simulink model "sim_pos_dist_obs_tcyb"  (R2020a)
settings: Solver=ode4  StartTime=0.0  StopTime=30.0  FixedStep=0.01  RelTol=1e-3
values from neighbouring files (symbols this model uses):
  alfa_theta = 20    [draw_compare_dist_pos_obs.m]
  alfa_theta_obs = 100    [draw_compare_dist_pos_obs.m]
  beta1 = 1.2    [draw_compare_dist_pos_obs.m]
  beta2 = 0.8    [draw_compare_dist_pos_obs.m]
  delta_p_i_0 = zeros(3, NF)    [draw_compare_dist_pos_obs.m]
  delta_v_i_0 = zeros(3, NF)    [draw_compare_dist_pos_obs.m]
  dp_aa_t = 0.2 * ones(3, 5) + ( 1.0 - 0.2 ) * rand(3, 5)    [draw_compare_dist_pos_obs.m]
  dp_ff_t = [ 0.4 * ones(1, 5) + ( 1.0 - 0.4 ) * rand(1, 5);                      0.4 * ones(1, 5) + ( 1.0 - 0.4 ) * rand(1, 5);                      0.2 * ones(1, 5) + ( 0.6 - 0.2 ) * rand(1, 5) ]    [draw_compare_dist_pos_obs.m]
  dp_phi_t = ( - pi / 2 ) * ones(3, 5) + ( pi / 2 - ( - pi / 2 ) ) * rand(3, 5)    [draw_compare_dist_pos_obs.m]
  eps_zeta = 0.2    [draw_compare_dist_pos_obs.m]
  etai_0 = zeros(3,5)    [draw_compare_dist_pos_obs.m]
  gamma_obs_1 = 4    [draw_compare_dist_pos_obs.m]
  gamma_obs_2 = 4    [draw_compare_dist_pos_obs.m]
  kai_1_t = 0.02    [draw_compare_dist_pos_obs.m]
  kai_3_t = 0.1    [draw_compare_dist_pos_obs.m]
  kai_chi_1 = diag([6; 6; 6])    [draw_compare_dist_pos_obs.m]
  kai_chi_2 = diag([6; 6; 6])    [draw_compare_dist_pos_obs.m]
  kai_u_1 = diag([8; 8; 8])    [draw_compare_dist_pos_obs.m]
  kai_u_2 = diag([8; 8; 8])    [draw_compare_dist_pos_obs.m]
  ksii_0 = zeros(3,5)    [draw_compare_dist_pos_obs.m]
  l1v = diag([20; 20; 20])    [draw_compare_dist_pos_obs.m]
  l2v = diag([30; 30; 30])    [draw_compare_dist_pos_obs.m]
  mass_i = zeros(1,NF)    [draw_compare_dist_pos_obs.m]
  Mii = diag([1;0;0;0;1])    [draw_compare_dist_pos_obs.m]
  pos0 = zeros(3, 1)    [draw_compare_dist_pos_obs.m]
  PZ0 = P0(3)    [draw_compare_dist_pos_obs.m]
  PZ1 = 10    [draw_compare_dist_pos_obs.m]
  Qci_init = repmat([1;0;0;0],1,NF)    [draw_compare_dist_pos_obs.m]
  R0 = 4    [draw_compare_dist_pos_obs.m]
  R1 = 8    [draw_compare_dist_pos_obs.m]
  Rx2 = 10    [draw_compare_dist_pos_obs.m]
  Ry2 = 6    [draw_compare_dist_pos_obs.m]
  Rz2 = 4    [draw_compare_dist_pos_obs.m]
  T0 = 0    [draw_compare_dist_pos_obs.m]
  T1 = tseq1    (= 10)    [draw_compare_dist_pos_obs.m]
  T12 = tseq1 + tseq12    (= 20)    [draw_compare_dist_pos_obs.m]
  T2 = tseq1 + tseq12 + tseq2    (= 30)    [draw_compare_dist_pos_obs.m]
  tf2_zeta = 2    [draw_compare_dist_pos_obs.m]
  theta0 = ( 2 / 5 ) * pi    (= 1.25663706144)    [draw_compare_dist_pos_obs.m]
  vel0 = zeros(3, 1)    [draw_compare_dist_pos_obs.m]
  Wij = [0,0,1,0,0;              0,0,1,1,0;              1,0,0,0,1;              0,1,1,0,0;              0,0,1,0,0]    [draw_compare_dist_pos_obs.m]
  X1 = 8    [draw_compare_dist_pos_obs.m]
  X2 = 2    [draw_compare_dist_pos_obs.m]
  X3 = 3    [draw_compare_dist_pos_obs.m]
  Y1 = 10    [draw_compare_dist_pos_obs.m]
  Y2 = 2    [draw_compare_dist_pos_obs.m]
  Y3 = 4    [draw_compare_dist_pos_obs.m]
  Z1 = 4    [draw_compare_dist_pos_obs.m]
  Z2 = -6    [draw_compare_dist_pos_obs.m]
  Z3 = 2    [draw_compare_dist_pos_obs.m]
undefined symbols (not defined in the file or in its folder): cal_frac_squ, p_beta1, p_beta2, p_dbeta1, p_dbeta2, p_gamma1_pos, p_gamma1_vel, p_gamma2_pos, p_gamma2_vel, q_beta1, q_beta2, q_dbeta1, q_dbeta2, q_gamma1_pos, q_gamma1_vel, q_gamma2_pos, q_gamma2_vel
(part 2 of 4)

== matlab function sim_pos_dist_obs_tcyb/choose ksi_est_err 19 ==
  data: x input; y output
function y = fcn(x)
iiuav = 5;
y = x(:,iiuav);

== matlab function sim_pos_dist_obs_tcyb/leader control input ==
  data: t input; u0 output; T1 input; T2 input; R0 input; R1 input; Rx2 input; Ry2 input; Rz2 input
function u0  = fcn(t, T1, T2, R0, R1, Rx2, Ry2, Rz2)
%%%% 给出领导者参考加速度控制输入
u0 = zeros(3, 1);

if t <= ( T1 + 1e-05 )
    u0(1, 1) = - ( 4 * pi * sin( ( 2 * pi * ( t - 0 ) ) / ( 0 - T1 ) ) * ( R0 - R1 ) ) / ( ( 0 - T1 ) ^ 2 ) ...
                        - ( 4 * ( pi ^ 2 ) * cos( ( 2 * pi * ( t - 0 ) ) / ( 0 - T1 ) ) ...
                        * ( R0 + ( ( R0 - R1 ) * ( t - 0 ) ) / ( 0 - T1 ) ) ) / ( ( 0 - T1 ) ^ 2 );
    u0(2, 1) = ( 4 * pi * cos( ( 2 * pi * ( t - 0 ) ) / ( 0 - T1 ) ) * ( R0 - R1 ) ) / ( ( 0 - T1 ) ^ 2 ) ...
                        - ( 4 * ( pi ^ 2 ) * sin( ( 2 * pi * ( t - 0 ) ) / ( 0 - T1 ) ) ...
                        * ( R0 + ( ( R0 - R1 ) * ( t - 0 ) ) / ( 0 - T1 ) ) ) / ( ( 0 - T1 ) ^ 2 );
    u0(3, 1) = 0;
else
    u0(1, 1) = ( 4 * Rx2 * ( pi ^ 2 ) * cos( ( 2 * pi * ( t - T1 ) ) / ( T1 - T2 ) ) ) / ( ( T1 - T2 ) ^ 2 );
    u0(2, 1) = - ( 16 * Ry2 * ( pi ^ 2 ) * sin( ( 4 * pi * ( t - T1 ) ) / ( T1 - T2 ) ) ) / ( ( T1 - T2 ) ^ 2 );
    u0(3, 1) = ( 16 * Rz2 * ( pi ^ 2 ) * sin( ( 4 * pi * ( t - T1 ) ) / ( T1 - T2 ) ) ) / ( ( T1 - T2 ) ^ 2 );
end

== matlab function sim_pos_dist_obs_tcyb/choose ksi_est_err 20 ==
  data: x input; y output
function y = fcn(x)
iiuav = 5;
y = x(:,iiuav);

== matlab function sim_pos_dist_obs_tcyb/trans to column18 ==
  data: x input; y output
function y = fcn(x)
y = x(:);

== matlab function sim_pos_dist_obs_tcyb/trans to column19 ==
  data: x input; y output
function y = fcn(x)
y = x(:);

== matlab function sim_pos_dist_obs_tcyb/cal dchi agent 1 ==
  data: kai_chi_1 input; d_chi_1 output; kai_chi_2 input; d_theta_err_ksi_1_vec input; d_theta_err_ksi_2_vec input
function d_chi_1 = fcn(kai_chi_1, kai_chi_2, d_theta_err_ksi_1_vec, d_theta_err_ksi_2_vec)
%%%% 固定时间虚拟速度控制量导数d_chi
iiuav = 1;
d_chi_1 = -kai_chi_1 * d_theta_err_ksi_1_vec(:,iiuav) - kai_chi_2 * d_theta_err_ksi_2_vec(:,iiuav);

== matlab function sim_pos_dist_obs_tcyb/combine dtheta_err_ksi ==
  data: d_theta_err_ksi_1_1 input; d_theta_err_ksi_1_2 input; d_theta_err_ksi_1_3 input; d_theta_err_ksi_1_4 input; d_theta_err_ksi_1_5 input; d_theta_err_ksi_1_vec output; d_theta_err_ksi_2_1 input; d_theta_err_ksi_2_vec output; d_theta_err_ksi_2_2 input; d_theta_err_ksi_2_3 input; d_theta_err_ksi_2_4 input; d_theta_err_ksi_2_5 input
function [d_theta_err_ksi_1_vec, d_theta_err_ksi_2_vec]  = fcn(d_theta_err_ksi_1_1, d_theta_err_ksi_1_2, d_theta_err_ksi_1_3, d_theta_err_ksi_1_4, d_theta_err_ksi_1_5, ...
                                                                                                                d_theta_err_ksi_2_1, d_theta_err_ksi_2_2, d_theta_err_ksi_2_3, d_theta_err_ksi_2_4, d_theta_err_ksi_2_5)
%%%% 合并平滑函数的导数
d_theta_err_ksi_1_vec = [d_theta_err_ksi_1_1(:), d_theta_err_ksi_1_2(:), d_theta_err_ksi_1_3(:), d_theta_err_ksi_1_4(:), d_theta_err_ksi_1_5(:)];
d_theta_err_ksi_2_vec = [d_theta_err_ksi_2_1(:), d_theta_err_ksi_2_2(:), d_theta_err_ksi_2_3(:), d_theta_err_ksi_2_4(:), d_theta_err_ksi_2_5(:)];

== matlab function sim_pos_dist_obs_tcyb/cal dchi agent 2 ==
  data: kai_chi_1 input; d_chi_2 output; kai_chi_2 input; d_theta_err_ksi_1_vec input; d_theta_err_ksi_2_vec input
function d_chi_2 = fcn(kai_chi_1, kai_chi_2, d_theta_err_ksi_1_vec, d_theta_err_ksi_2_vec)
%%%% 固定时间虚拟速度控制量导数d_chi
iiuav = 2;
d_chi_2 = -kai_chi_1 * d_theta_err_ksi_1_vec(:,iiuav) - kai_chi_2 * d_theta_err_ksi_2_vec(:,iiuav);

== matlab function sim_pos_dist_obs_tcyb/cal dchi agent 3 ==
  data: kai_chi_1 input; d_chi_3 output; kai_chi_2 input; d_theta_err_ksi_1_vec input; d_theta_err_ksi_2_vec input
function d_chi_3 = fcn(kai_chi_1, kai_chi_2, d_theta_err_ksi_1_vec, d_theta_err_ksi_2_vec)
%%%% 固定时间虚拟速度控制量导数d_chi
iiuav = 3;
d_chi_3 = -kai_chi_1 * d_theta_err_ksi_1_vec(:,iiuav) - kai_chi_2 * d_theta_err_ksi_2_vec(:,iiuav);

== matlab function sim_pos_dist_obs_tcyb/cal dchi agent 4 ==
  data: kai_chi_1 input; d_chi_4 output; kai_chi_2 input; d_theta_err_ksi_1_vec input; d_theta_err_ksi_2_vec input
function d_chi_4 = fcn(kai_chi_1, kai_chi_2, d_theta_err_ksi_1_vec, d_theta_err_ksi_2_vec)
%%%% 固定时间虚拟速度控制量导数d_chi
iiuav = 4;
d_chi_4 = -kai_chi_1 * d_theta_err_ksi_1_vec(:,iiuav) - kai_chi_2 * d_theta_err_ksi_2_vec(:,iiuav);

== matlab function sim_pos_dist_obs_tcyb/cal dchi agent 5 ==
  data: kai_chi_1 input; d_chi_5 output; kai_chi_2 input; d_theta_err_ksi_1_vec input; d_theta_err_ksi_2_vec input
function d_chi_5 = fcn(kai_chi_1, kai_chi_2, d_theta_err_ksi_1_vec, d_theta_err_ksi_2_vec)
%%%% 固定时间虚拟速度控制量导数d_chi
iiuav = 5;
d_chi_5 = -kai_chi_1 * d_theta_err_ksi_1_vec(:,iiuav) - kai_chi_2 * d_theta_err_ksi_2_vec(:,iiuav);

== matlab function sim_pos_dist_obs_tcyb/combine dchi ==
  data: d_chi_1 input; d_chi_2 input; d_chi_3 input; d_chi_4 input; d_chi_5 input; d_chi_vec output
function d_chi_vec  = fcn(d_chi_1, d_chi_2, d_chi_3, d_chi_4, d_chi_5)
%%%% 合并领导者位置观测器输出结果
d_chi_vec = [d_chi_1(:), d_chi_2(:), d_chi_3(:), d_chi_4(:), d_chi_5(:)];

== matlab function sim_pos_dist_obs_tcyb/cal x1_hat agent 4 ==
  data: gamma_obs_1 input; zeta2 input; d_x1_hat_4 output; dzeta2 input; x2_hat_vec input; x1_tilt_vec input
function d_x1_hat_4 = fcn(gamma_obs_1, zeta2, dzeta2, x2_hat_vec, x1_tilt_vec)
%%%% 计算状态观测误差
iiuav = 4;
d_x1_hat_4 = x2_hat_vec(:,iiuav) + gamma_obs_1 * zeta2 * x1_tilt_vec(:,iiuav) + ( 2 * dzeta2 / zeta2 ) * x1_tilt_vec(:,iiuav);

== matlab function sim_pos_dist_obs_tcyb/cal x1_hat agent 5 ==
  data: gamma_obs_1 input; zeta2 input; d_x1_hat_5 output; dzeta2 input; x2_hat_vec input; x1_tilt_vec input
function d_x1_hat_5 = fcn(gamma_obs_1, zeta2, dzeta2, x2_hat_vec, x1_tilt_vec)
%%%% 计算状态观测误差
iiuav = 5;
d_x1_hat_5 = x2_hat_vec(:,iiuav) + gamma_obs_1 * zeta2 * x1_tilt_vec(:,iiuav) + ( 2 * dzeta2 / zeta2 ) * x1_tilt_vec(:,iiuav);

== matlab function sim_pos_dist_obs_tcyb/cal x1_tilt ==
  data: ksi_i_vec input; x1_hat_vec input; x1_tilt_vec output
function x1_tilt_vec = fcn(ksi_i_vec, x1_hat_vec)
%%%% 计算状态观测误差
x1_tilt_vec = zeros(3,5);
for iiuav = 1:5
    x1_tilt_vec(:,iiuav) = ksi_i_vec(:,iiuav) - x1_hat_vec(:,iiuav);
end

== matlab function sim_pos_dist_obs_tcyb/cal x2_hat agent 2 ==
  data: gamma_obs_2 input; zeta2 input; d_x2_hat_2 output; dzeta2 input; Ri input; ui input; dp_hat_vec input; x1_tilt_vec input
function d_x2_hat_2 = fcn(gamma_obs_2, zeta2, dzeta2, Ri, ui, dp_hat_vec, x1_tilt_vec)
%%%% 计算状态观测误差
iiuav = 2;
g0 = 9.80663;
e3 = [0;0;1];
d_x2_hat_2 = dp_hat_vec(:,iiuav) + gamma_obs_2 * (zeta2 ^ 2) * x1_tilt_vec(:,iiuav) ...
                                                                + ( dzeta2 / zeta2 ) * x1_tilt_vec(:,iiuav) ...
                                                                - g0 * e3 + norm(ui(:,iiuav),2) * Ri(:,:,iiuav) * e3;

== matlab function sim_pos_dist_obs_tcyb/generate translational disturbance agent 5 ==
  data: dp_aa_t input; dp_ff_t input; dp_phi_t input; dp_5 output; t input
function dp_5 = fcn(dp_aa_t, dp_ff_t, dp_phi_t, t)
%%%% 平移动力学方程中的扰动项设置
epsil_t = zeros(3, 1);

for kk = 1:5
    epsil_t = epsil_t + dp_aa_t(:, kk) .* sin( 2 * pi * dp_ff_t(:, kk) * t + dp_phi_t(:, kk) );
end

dp_5 = [ epsil_t(1) + 1.6 * sin( 0.2 * t ) + 2.0 * cos( 0.3 * t ) + 1.4 * sin( 0.5 * t ) ...
                + 4 * exp( -0.1 * t ) * sin( 0.5 * t ) + 3 / ( 1 + exp( -0.2 * ( t - 15 ) ) ); ...
                epsil_t(2) + 1.2 * sin( 0.1 * t ) + 3 * cos( 0.2 * t ) + 0.8 * sin( 0.4 * t ) ...
                + 2 * exp( -0.15 * t ) * cos( 0.6 * t ) + 3 / ( 1 + exp( -0.3 * ( t - 25 ) ) ); ...
                epsil_t(3) + 1.8 * sin( 0.1 * t ) + 1.6 * sin( 0.2 * t ) + 1.6 * cos( 0.3 * t ) ...
                + 4 * exp( -0.05 * t ) * sin( 0.4 * t + pi / 4 ) + 3 / ( 1 + exp( -0.5 * ( t - 20 ) ) ) ];

== matlab function sim_pos_dist_obs_tcyb/cal x2_hat agent 3 ==
  data: gamma_obs_2 input; zeta2 input; d_x2_hat_3 output; dzeta2 input; Ri input; ui input; dp_hat_vec input; x1_tilt_vec input
function d_x2_hat_3 = fcn(gamma_obs_2, zeta2, dzeta2, Ri, ui, dp_hat_vec, x1_tilt_vec)
%%%% 计算状态观测误差
iiuav = 3;
g0 = 9.80663;
e3 = [0;0;1];
d_x2_hat_3 = dp_hat_vec(:,iiuav) + gamma_obs_2 * (zeta2 ^ 2) * x1_tilt_vec(:,iiuav) ...
                                                                + ( dzeta2 / zeta2 ) * x1_tilt_vec(:,iiuav) ...
                                                                - g0 * e3 + norm(ui(:,iiuav),2) * Ri(:,:,iiuav) * e3;

== matlab function sim_pos_dist_obs_tcyb/cal x2_hat agent 4 ==
  data: gamma_obs_2 input; zeta2 input; d_x2_hat_4 output; dzeta2 input; Ri input; ui input; dp_hat_vec input; x1_tilt_vec input
function d_x2_hat_4 = fcn(gamma_obs_2, zeta2, dzeta2, Ri, ui, dp_hat_vec, x1_tilt_vec)
%%%% 计算状态观测误差
iiuav = 4;
g0 = 9.80663;
e3 = [0;0;1];
d_x2_hat_4 = dp_hat_vec(:,iiuav) + gamma_obs_2 * (zeta2 ^ 2) * x1_tilt_vec(:,iiuav) ...
                                                                + ( dzeta2 / zeta2 ) * x1_tilt_vec(:,iiuav) ...
                                                                - g0 * e3 + norm(ui(:,iiuav),2) * Ri(:,:,iiuav) * e3;

== matlab function sim_pos_dist_obs_tcyb/cal dp_hat agent 2 ==
  data: gamma_obs_3 input; zeta2 input; d_dp_hat_2 output; x1_tilt_vec input
function d_dp_hat_2 = fcn(gamma_obs_3, zeta2, x1_tilt_vec)
%%%% 计算状态观测误差
iiuav = 2;
d_dp_hat_2 = gamma_obs_3 * (zeta2 ^ 3) * x1_tilt_vec(:,iiuav);

== matlab function sim_pos_dist_obs_tcyb/cal dp_hat agent 3 ==
  data: gamma_obs_3 input; zeta2 input; d_dp_hat_3 output; x1_tilt_vec input
function d_dp_hat_3 = fcn(gamma_obs_3, zeta2, x1_tilt_vec)
%%%% 计算状态观测误差
iiuav = 3;
d_dp_hat_3 = gamma_obs_3 * (zeta2 ^ 3) * x1_tilt_vec(:,iiuav);

== matlab function sim_pos_dist_obs_tcyb/cal dp_hat agent 4 ==
  data: gamma_obs_3 input; zeta2 input; d_dp_hat_4 output; x1_tilt_vec input
function d_dp_hat_4 = fcn(gamma_obs_3, zeta2, x1_tilt_vec)
%%%% 计算状态观测误差
iiuav = 4;
d_dp_hat_4 = gamma_obs_3 * (zeta2 ^ 3) * x1_tilt_vec(:,iiuav);

== matlab function sim_pos_dist_obs_tcyb/cal dp_hat agent 5 ==
  data: gamma_obs_3 input; zeta2 input; d_dp_hat_5 output; x1_tilt_vec input
function d_dp_hat_5 = fcn(gamma_obs_3, zeta2, x1_tilt_vec)
%%%% 计算状态观测误差
iiuav = 5;
d_dp_hat_5 = gamma_obs_3 * (zeta2 ^ 3) * x1_tilt_vec(:,iiuav);

== matlab function sim_pos_dist_obs_tcyb/cal x2_hat agent 5 ==
  data: gamma_obs_2 input; zeta2 input; d_x2_hat_5 output; dzeta2 input; Ri input; ui input; dp_hat_vec input; x1_tilt_vec input
function d_x2_hat_5 = fcn(gamma_obs_2, zeta2, dzeta2, Ri, ui, dp_hat_vec, x1_tilt_vec)
%%%% 计算状态观测误差
iiuav = 5;
g0 = 9.80663;
e3 = [0;0;1];
d_x2_hat_5 = dp_hat_vec(:,iiuav) + gamma_obs_2 * (zeta2 ^ 2) * x1_tilt_vec(:,iiuav) ...
                                                                + ( dzeta2 / zeta2 ) * x1_tilt_vec(:,iiuav) ...
                                                                - g0 * e3 + norm(ui(:,iiuav),2) * Ri(:,:,iiuav) * e3;

== matlab function sim_pos_dist_obs_tcyb/cal zeta0 zeta2 dzeta2 d2zeta2 ==
  data: tsim input; tf2_zeta input; zeta2 output; eps_zeta input; dzeta2 output
function [zeta2, dzeta2] = fcn(tsim, tf2_zeta, eps_zeta)
%%%% 计算预设时间函数

if tsim <= 0
    zeta0_t = 0;
    d_zeta0_t = 0;
else
    zeta0_t = exp(-1/tsim);
    d_zeta0_t = (1/(tsim^2)) * exp(-1/tsim);
end

if tf2_zeta - tsim <= 0
    zeta0_tf_t = 0;
    d_zeta0_tf_t = 0;
else
    zeta0_tf_t = exp(-1/(tf2_zeta - tsim));
    d_zeta0_tf_t = -(1/((tf2_zeta - tsim)^2)) * exp(-1/(tf2_zeta - tsim));
end

zeta2 = ( zeta0_tf_t + zeta0_t ) / ( (1 + eps_zeta) * zeta0_tf_t + eps_zeta * zeta0_t );
dzeta2 = ( d_zeta0_t * zeta0_tf_t - zeta0_t * d_zeta0_tf_t ) / ( ( (1+eps_zeta) * zeta0_tf_t + eps_zeta * zeta0_t ) ^2 );

== matlab function sim_pos_dist_obs_tcyb/cal Rei ==
  data: Rei output; Qei input
function Rei = fcn(Qei)
%%%% 使用罗德里格公式由四元数Qei求解Rei
Rei = zeros(3,3,5);
for iuav = 1:5
    thetaei_tmp = Qei(1,iuav);
    qei_tmp = Qei(2:4,iuav);
    Rei(:,:,iuav) = ((thetaei_tmp^2) - (qei_tmp')*qei_tmp) * eye(3,3) ...
                            + 2 * qei_tmp * (qei_tmp') ...
                            - 2 * thetaei_tmp * cal_askew_mat(qei_tmp);
end

end

== matlab function sim_pos_dist_obs_tcyb/depart Re5 ==
  data: y output; x input
function y = fcn(x)
y = x(:,:,5);

end

== matlab function sim_pos_dist_obs_tcyb/combine translational disturbance ==
  data: dp_vec output; dp_1 input; dp_2 input; dp_3 input; dp_4 input; dp_5 input
function dp_vec = fcn(dp_1, dp_2, dp_3, dp_4, dp_5)
%%%% 合并领导者编队跟踪误差结果
dp_vec = [dp_1(:), dp_2(:), dp_3(:), dp_4(:), dp_5(:)];

== matlab function sim_pos_dist_obs_tcyb/depart Re1 ==
  data: y output; x input
function y = fcn(x)
y = x(:,:,1);

end

== matlab function sim_pos_dist_obs_tcyb/depart Re2 ==
  data: y output; x input
function y = fcn(x)
y = x(:,:,2);

end

== matlab function sim_pos_dist_obs_tcyb/depart Re3 ==
  data: y output; x input
function y = fcn(x)
y = x(:,:,3);

end

== matlab function sim_pos_dist_obs_tcyb/depart Re4 ==
  data: y output; x input
function y = fcn(x)
y = x(:,:,4);

end

== matlab function sim_pos_dist_obs_tcyb/choose ksi_est_err 1 ==
  data: x input; y output
function y = fcn(x)
iiuav = 1;
y = x(:,iiuav);

== matlab function sim_pos_dist_obs_tcyb/trans to column35 ==
  data: x input; y output
function y = fcn(x)
y = x(:);

== matlab function sim_pos_dist_obs_tcyb/cal Rci from ui ==
  data: Rci output; mi input; ui input
function Rci = fcn(mi, ui)
Rci = zeros(3,3,5);
for iiuav = 1:5
    Rci(:,:,iiuav) = cal_Rc_with_u(mi(iiuav), ui(:,iiuav));
end

end

== matlab function sim_pos_dist_obs_tcyb/cal x1_hat agent 1 ==
  data: gamma_obs_1 input; zeta2 input; d_x1_hat_1 output; dzeta2 input; x2_hat_vec input; x1_tilt_vec input
function d_x1_hat_1 = fcn(gamma_obs_1, zeta2, dzeta2, x2_hat_vec, x1_tilt_vec)
%%%% 计算状态观测误差
iiuav = 1;
d_x1_hat_1 = x2_hat_vec(:,iiuav) + gamma_obs_1 * zeta2 * x1_tilt_vec(:,iiuav) + ( 2 * dzeta2 / zeta2 ) * x1_tilt_vec(:,iiuav);

== matlab function sim_pos_dist_obs_tcyb/combine x1_hat ==
  data: x1_hat_1 input; x1_hat_2 input; x1_hat_3 input; x1_hat_4 input; x1_hat_5 input; x1_hat_vec output
function x1_hat_vec  = fcn(x1_hat_1, x1_hat_2, x1_hat_3, x1_hat_4, x1_hat_5)
%%%% 合并领导者位置观测器输出结果
x1_hat_vec = [x1_hat_1(:), x1_hat_2(:), x1_hat_3(:), x1_hat_4(:), x1_hat_5(:)];

== matlab function sim_pos_dist_obs_tcyb/cal x2_hat agent 1 ==
  data: gamma_obs_2 input; zeta2 input; d_x2_hat_1 output; dzeta2 input; Ri input; ui input; dp_hat_vec input; x1_tilt_vec input
function d_x2_hat_1 = fcn(gamma_obs_2, zeta2, dzeta2, Ri, ui, dp_hat_vec, x1_tilt_vec)
%%%% 计算状态观测误差
iiuav = 1;
g0 = 9.80663;
e3 = [0;0;1];
d_x2_hat_1 = dp_hat_vec(:,iiuav) + gamma_obs_2 * (zeta2 ^ 2) * x1_tilt_vec(:,iiuav) ...
                                                                + ( dzeta2 / zeta2 ) * x1_tilt_vec(:,iiuav) ...
                                                                - g0 * e3 + norm(ui(:,iiuav),2) * Ri(:,:,iiuav) * e3;

== matlab function sim_pos_dist_obs_tcyb/combine x2_hat ==
  data: x2_hat_1 input; x2_hat_2 input; x2_hat_3 input; x2_hat_4 input; x2_hat_5 input; x2_hat_vec output
function x2_hat_vec  = fcn(x2_hat_1, x2_hat_2, x2_hat_3, x2_hat_4, x2_hat_5)
%%%% 合并领导者位置观测器输出结果
x2_hat_vec = [x2_hat_1(:), x2_hat_2(:), x2_hat_3(:), x2_hat_4(:), x2_hat_5(:)];

== matlab function sim_pos_dist_obs_tcyb/cal dp_hat agent 1 ==
  data: gamma_obs_3 input; zeta2 input; d_dp_hat_1 output; x1_tilt_vec input
function d_dp_hat_1 = fcn(gamma_obs_3, zeta2, x1_tilt_vec)
%%%% 计算状态观测误差
iiuav = 1;
d_dp_hat_1 = gamma_obs_3 * (zeta2 ^ 3) * x1_tilt_vec(:,iiuav);

== matlab function sim_pos_dist_obs_tcyb/combine dp_hat ==
  data: dp_hat_1 input; dp_hat_2 input; dp_hat_3 input; dp_hat_4 input; dp_hat_5 input; dp_hat_vec output
function dp_hat_vec  = fcn(dp_hat_1, dp_hat_2, dp_hat_3, dp_hat_4, dp_hat_5)
%%%% 合并扰动观测值dp_hat
dp_hat_vec = [dp_hat_1(:), dp_hat_2(:), dp_hat_3(:), dp_hat_4(:), dp_hat_5(:)];

== matlab function sim_pos_dist_obs_tcyb/cal abs 2 ==
  data: x input; y output
function y = fcn(x)
y = abs(x(:));

== matlab function sim_pos_dist_obs_tcyb/cal abs 31 ==
  data: x input; y output
function y = fcn(x)
y = abs(x(:));

== matlab function sim_pos_dist_obs_tcyb/cal abs 32 ==
  data: x input; y output
function y = fcn(x)
y = abs(x(:));

== matlab function sim_pos_dist_obs_tcyb/cal theta_phi agent 1 ==
  data: alfa_theta input; phi_squ_1_1 input; theta_phi_1_1 output; phi_squ_2_1 input; phi_vec input; theta_phi_2_1 output
function [theta_phi_1_1, theta_phi_2_1] = fcn(alfa_theta, phi_squ_1_1, phi_squ_2_1, phi_vec)
%%%% 计算平滑递增函数
iiuav = 1;
theta_phi_1_1 = phi_squ_1_1(:) .* ( -1 + 2 ./ ( 1 + exp( -alfa_theta .* phi_vec(:,iiuav) ) ) );
theta_phi_2_1 = phi_squ_2_1(:) .* ( -1 + 2 ./ ( 1 + exp( -alfa_theta .* phi_vec(:,iiuav) ) ) );

== matlab function sim_pos_dist_obs_tcyb/choose ksi_est_err 31 ==
  data: x input; y output
function y = fcn(x)
iiuav = 1;
y = x(:,iiuav);

== matlab function sim_pos_dist_obs_tcyb/choose ksi_est_err 32 ==
  data: x input; y output
function y = fcn(x)
iiuav = 1;
y = x(:,iiuav);

== matlab function sim_pos_dist_obs_tcyb/trans to column30 ==
  data: x input; y output
function y = fcn(x)
y = x(:);

== matlab function sim_pos_dist_obs_tcyb/trans to column31 ==
  data: x input; y output
function y = fcn(x)
y = x(:);

== matlab function sim_pos_dist_obs_tcyb/cal abs 33 ==
  data: x input; y output
function y = fcn(x)
y = abs(x(:));

== matlab function sim_pos_dist_obs_tcyb/cal abs 34 ==
  data: x input; y output
function y = fcn(x)
y = abs(x(:));

== matlab function sim_pos_dist_obs_tcyb/cal theta_err_ksi agent 1 ==
  data: alfa_theta input; err_ksi_squ_1_node_1 input; theta_err_ksi_1_1 output; err_ksi_squ_2_node_1 input; err_ksi_vec input; theta_err_ksi_2_1 output
function [theta_err_ksi_1_1, theta_err_ksi_2_1] = fcn(alfa_theta, err_ksi_squ_1_node_1, err_ksi_squ_2_node_1, err_ksi_vec)
%%%% 计算平滑递增函数
iiuav = 1;
theta_err_ksi_1_1 = err_ksi_squ_1_node_1(:) .* ( -1 + 2 ./ ( 1 + exp( -alfa_theta .* err_ksi_vec(:,iiuav) ) ) );
theta_err_ksi_2_1 = err_ksi_squ_2_node_1(:) .* ( -1 + 2 ./ ( 1 + exp( -alfa_theta .* err_ksi_vec(:,iiuav) ) ) );

== matlab function sim_pos_dist_obs_tcyb/cal theta_phi agent 2 ==
  data: alfa_theta input; phi_squ_1_2 input; theta_phi_1_2 output; phi_squ_2_2 input; phi_vec input; theta_phi_2_2 output
function [theta_phi_1_2, theta_phi_2_2] = fcn(alfa_theta, phi_squ_1_2, phi_squ_2_2, phi_vec)
%%%% 计算平滑递增函数
iiuav = 2;
theta_phi_1_2 = phi_squ_1_2(:) .* ( -1 + 2 ./ ( 1 + exp( -alfa_theta .* phi_vec(:,iiuav) ) ) );
theta_phi_2_2 = phi_squ_2_2(:) .* ( -1 + 2 ./ ( 1 + exp( -alfa_theta .* phi_vec(:,iiuav) ) ) );

== matlab function sim_pos_dist_obs_tcyb/choose ksi_est_err 33 ==
  data: x input; y output
function y = fcn(x)
iiuav = 2;
y = x(:,iiuav);

== matlab function sim_pos_dist_obs_tcyb/choose ksi_est_err 34 ==
  data: x input; y output
function y = fcn(x)
iiuav = 2;
y = x(:,iiuav);

== matlab function sim_pos_dist_obs_tcyb/trans to column32 ==
  data: x input; y output
function y = fcn(x)
y = x(:);

== matlab function sim_pos_dist_obs_tcyb/trans to column33 ==
  data: x input; y output
function y = fcn(x)
y = x(:);

== matlab function sim_pos_dist_obs_tcyb/cal abs 35 ==
  data: x input; y output
function y = fcn(x)
y = abs(x(:));

== matlab function sim_pos_dist_obs_tcyb/cal abs 36 ==
  data: x input; y output
function y = fcn(x)
y = abs(x(:));

== matlab function sim_pos_dist_obs_tcyb/cal theta_phi agent 3 ==
  data: alfa_theta input; phi_squ_1_3 input; theta_phi_1_3 output; phi_squ_2_3 input; phi_vec input; theta_phi_2_3 output
function [theta_phi_1_3, theta_phi_2_3] = fcn(alfa_theta, phi_squ_1_3, phi_squ_2_3, phi_vec)
%%%% 计算平滑递增函数
iiuav = 3;
theta_phi_1_3 = phi_squ_1_3(:) .* ( -1 + 2 ./ ( 1 + exp( -alfa_theta .* phi_vec(:,iiuav) ) ) );
theta_phi_2_3 = phi_squ_2_3(:) .* ( -1 + 2 ./ ( 1 + exp( -alfa_theta .* phi_vec(:,iiuav) ) ) );

== matlab function sim_pos_dist_obs_tcyb/choose ksi_est_err 35 ==
  data: x input; y output
function y = fcn(x)
iiuav = 3;
y = x(:,iiuav);

== matlab function sim_pos_dist_obs_tcyb/choose ksi_est_err 36 ==
  data: x input; y output
function y = fcn(x)
iiuav = 3;
y = x(:,iiuav);

== matlab function sim_pos_dist_obs_tcyb/trans to column34 ==
  data: x input; y output
function y = fcn(x)
y = x(:);

== matlab function sim_pos_dist_obs_tcyb/trans to column36 ==
  data: x input; y output
function y = fcn(x)
y = x(:);

== matlab function sim_pos_dist_obs_tcyb/cal abs 37 ==
  data: x input; y output
function y = fcn(x)
y = abs(x(:));

== matlab function sim_pos_dist_obs_tcyb/cal abs 38 ==
  data: x input; y output
function y = fcn(x)
y = abs(x(:));

== matlab function sim_pos_dist_obs_tcyb/trans to column1 ==
  data: x input; y output
function y = fcn(x)
y = x(:);

== matlab function sim_pos_dist_obs_tcyb/cal theta_phi agent 4 ==
  data: alfa_theta input; phi_squ_1_4 input; theta_phi_1_4 output; phi_squ_2_4 input; phi_vec input; theta_phi_2_4 output
function [theta_phi_1_4, theta_phi_2_4] = fcn(alfa_theta, phi_squ_1_4, phi_squ_2_4, phi_vec)
%%%% 计算平滑递增函数
iiuav = 4;
theta_phi_1_4 = phi_squ_1_4(:) .* ( -1 + 2 ./ ( 1 + exp( -alfa_theta .* phi_vec(:,iiuav) ) ) );
theta_phi_2_4 = phi_squ_2_4(:) .* ( -1 + 2 ./ ( 1 + exp( -alfa_theta .* phi_vec(:,iiuav) ) ) );

== matlab function sim_pos_dist_obs_tcyb/choose ksi_est_err 37 ==
  data: x input; y output
function y = fcn(x)
iiuav = 4;
y = x(:,iiuav);

== matlab function sim_pos_dist_obs_tcyb/choose ksi_est_err 38 ==
  data: x input; y output
function y = fcn(x)
iiuav = 4;
y = x(:,iiuav);

== matlab function sim_pos_dist_obs_tcyb/trans to column37 ==
  data: x input; y output
function y = fcn(x)
y = x(:);

== matlab function sim_pos_dist_obs_tcyb/trans to column38 ==
  data: x input; y output
function y = fcn(x)
y = x(:);

== matlab function sim_pos_dist_obs_tcyb/cal abs 39 ==
  data: x input; y output
function y = fcn(x)
y = abs(x(:));

== matlab function sim_pos_dist_obs_tcyb/cal abs 40 ==
  data: x input; y output
function y = fcn(x)
y = abs(x(:));

== matlab function sim_pos_dist_obs_tcyb/cal theta_phi agent 5 ==
  data: alfa_theta input; phi_squ_1_5 input; theta_phi_1_5 output; phi_squ_2_5 input; phi_vec input; theta_phi_2_5 output
function [theta_phi_1_5, theta_phi_2_5] = fcn(alfa_theta, phi_squ_1_5, phi_squ_2_5, phi_vec)
%%%% 计算平滑递增函数
iiuav = 5;
theta_phi_1_5 = phi_squ_1_5(:) .* ( -1 + 2 ./ ( 1 + exp( -alfa_theta .* phi_vec(:,iiuav) ) ) );
theta_phi_2_5 = phi_squ_2_5(:) .* ( -1 + 2 ./ ( 1 + exp( -alfa_theta .* phi_vec(:,iiuav) ) ) );

== matlab function sim_pos_dist_obs_tcyb/choose ksi_est_err 39 ==
  data: x input; y output
function y = fcn(x)
iiuav = 5;
y = x(:,iiuav);

== matlab function sim_pos_dist_obs_tcyb/cal abs 3 ==
  data: x input; y output
function y = fcn(x)
y = abs(x(:));

== matlab function sim_pos_dist_obs_tcyb/choose ksi_est_err 40 ==
  data: x input; y output
function y = fcn(x)
iiuav = 5;
y = x(:,iiuav);

== matlab function sim_pos_dist_obs_tcyb/trans to column39 ==
  data: x input; y output
function y = fcn(x)
y = x(:);

== matlab function sim_pos_dist_obs_tcyb/trans to column40 ==
  data: x input; y output
function y = fcn(x)
y = x(:);

== matlab function sim_pos_dist_obs_tcyb/combine theta_err_ksi1 ==
  data: theta_phi_1_1 input; theta_phi_1_2 input; theta_phi_1_3 input; theta_phi_1_4 input; theta_phi_1_5 input; theta_phi_1_vec output; theta_phi_2_1 input; theta_phi_2_vec output; theta_phi_2_2 input; theta_phi_2_3 input; theta_phi_2_4 input; theta_phi_2_5 input
function [theta_phi_1_vec, theta_phi_2_vec]  = fcn(theta_phi_1_1, theta_phi_1_2, theta_phi_1_3, theta_phi_1_4, theta_phi_1_5, ...
                                                                                            theta_phi_2_1, theta_phi_2_2, theta_phi_2_3, theta_phi_2_4, theta_phi_2_5)
%%%% 合并领导者位置观测器输出结果
theta_phi_1_vec = [theta_phi_1_1(:), theta_phi_1_2(:), theta_phi_1_3(:), theta_phi_1_4(:), theta_phi_1_5(:)];
theta_phi_2_vec = [theta_phi_2_1(:), theta_phi_2_2(:), theta_phi_2_3(:), theta_phi_2_4(:), theta_phi_2_5(:)];

== matlab function sim_pos_dist_obs_tcyb/cal ui agent 1 ==
  data: kai_u_1 input; ui_1 output; kai_u_2 input; d_chi_vec input; theta_phi_1_vec input; theta_phi_2_vec input; dp_hat_vec input
function ui_1 = fcn(kai_u_1, kai_u_2, d_chi_vec, theta_phi_1_vec, theta_phi_2_vec, dp_hat_vec)
%%%% 计算控制输入ui
iiuav = 1;
g0 = 9.80663;
e3 = [0;0;1];
ui_1 = g0 * e3 + d_chi_vec(:,iiuav) - kai_u_1 * theta_phi_1_vec(:,iiuav) - kai_u_2 * theta_phi_2_vec(:,iiuav) - dp_hat_vec(:,iiuav);

== matlab function sim_pos_dist_obs_tcyb/cal ui agent 2 ==
  data: kai_u_1 input; ui_2 output; kai_u_2 input; d_chi_vec input; theta_phi_1_vec input; theta_phi_2_vec input; dp_hat_vec input
function ui_2 = fcn(kai_u_1, kai_u_2, d_chi_vec, theta_phi_1_vec, theta_phi_2_vec, dp_hat_vec)
%%%% 计算控制输入ui
iiuav = 2;
g0 = 9.80663;
e3 = [0;0;1];
ui_2 = g0 * e3 + d_chi_vec(:,iiuav) - kai_u_1 * theta_phi_1_vec(:,iiuav) - kai_u_2 * theta_phi_2_vec(:,iiuav) - dp_hat_vec(:,iiuav);

== matlab function sim_pos_dist_obs_tcyb/cal ui agent 3 ==
  data: kai_u_1 input; ui_3 output; kai_u_2 input; d_chi_vec input; theta_phi_1_vec input; theta_phi_2_vec input; dp_hat_vec input
function ui_3 = fcn(kai_u_1, kai_u_2, d_chi_vec, theta_phi_1_vec, theta_phi_2_vec, dp_hat_vec)
%%%% 计算控制输入ui
iiuav = 3;
g0 = 9.80663;
e3 = [0;0;1];
ui_3 = g0 * e3 + d_chi_vec(:,iiuav) - kai_u_1 * theta_phi_1_vec(:,iiuav) - kai_u_2 * theta_phi_2_vec(:,iiuav) - dp_hat_vec(:,iiuav);

== matlab function sim_pos_dist_obs_tcyb/cal abs 4 ==
  data: x input; y output
function y = fcn(x)
y = abs(x(:));

== matlab function sim_pos_dist_obs_tcyb/cal ui agent 4 ==
  data: kai_u_1 input; ui_4 output; kai_u_2 input; d_chi_vec input; theta_phi_1_vec input; theta_phi_2_vec input; dp_hat_vec input
function ui_4 = fcn(kai_u_1, kai_u_2, d_chi_vec, theta_phi_1_vec, theta_phi_2_vec, dp_hat_vec)
%%%% 计算控制输入ui
iiuav = 4;
g0 = 9.80663;
e3 = [0;0;1];
ui_4 = g0 * e3 + d_chi_vec(:,iiuav) - kai_u_1 * theta_phi_1_vec(:,iiuav) - kai_u_2 * theta_phi_2_vec(:,iiuav) - dp_hat_vec(:,iiuav);

== matlab function sim_pos_dist_obs_tcyb/cal ui agent 5 ==
  data: kai_u_1 input; ui_5 output; kai_u_2 input; d_chi_vec input; theta_phi_1_vec input; theta_phi_2_vec input; dp_hat_vec input
function ui_5 = fcn(kai_u_1, kai_u_2, d_chi_vec, theta_phi_1_vec, theta_phi_2_vec, dp_hat_vec)
%%%% 计算控制输入ui
iiuav = 5;
g0 = 9.80663;
e3 = [0;0;1];
ui_5 = g0 * e3 + d_chi_vec(:,iiuav) - kai_u_1 * theta_phi_1_vec(:,iiuav) - kai_u_2 * theta_phi_2_vec(:,iiuav) - dp_hat_vec(:,iiuav);

== matlab function sim_pos_dist_obs_tcyb/combine ui ==
  data: ui_1 input; ui_2 input; ui_3 input; ui_4 input; ui_5 input; ui output
function ui  = fcn(ui_1, ui_2, ui_3, ui_4, ui_5)
%%%% 合并控制输入ui
ui = [ui_1(:), ui_2(:), ui_3(:), ui_4(:), ui_5(:)];

== matlab function sim_pos_dist_obs_tcyb/cal disturbance observation error dp_tilt ==
  data: dp_vec input; dp_tilt_vec output; dp_hat_vec input
function dp_tilt_vec = fcn(dp_vec, dp_hat_vec)
%%%% 计算扰动观测器估计误差dp_tilt
dp_tilt_vec = zeros(3,5);
for iiuav = 1:5
    dp_tilt_vec(:,iiuav) = dp_vec(:,iiuav) - dp_hat_vec(:,iiuav);
end

== matlab function sim_pos_dist_obs_tcyb/cal abs 41 ==
  data: x input; y output
function y = fcn(x)
y = abs(x(:));

== matlab function sim_pos_dist_obs_tcyb/cal abs 42 ==
  data: x input; y output
function y = fcn(x)
y = abs(x(:));

== matlab function sim_pos_dist_obs_tcyb/cal abs 43 ==
  data: x input; y output
function y = fcn(x)
y = abs(x(:));

== matlab function sim_pos_dist_obs_tcyb/cal theta_err_ksi agent 2 ==
  data: alfa_theta input; err_ksi_squ_1_node_2 input; theta_err_ksi_1_2 output; err_ksi_squ_2_node_2 input; err_ksi_vec input; theta_err_ksi_2_2 output
function [theta_err_ksi_1_2, theta_err_ksi_2_2] = fcn(alfa_theta, err_ksi_squ_1_node_2, err_ksi_squ_2_node_2, err_ksi_vec)
%%%% 计算平滑递增函数
iiuav = 2;
theta_err_ksi_1_2 = err_ksi_squ_1_node_2(:) .* ( -1 + 2 ./ ( 1 + exp( -alfa_theta .* err_ksi_vec(:,iiuav) ) ) );
theta_err_ksi_2_2 = err_ksi_squ_2_node_2(:) .* ( -1 + 2 ./ ( 1 + exp( -alfa_theta .* err_ksi_vec(:,iiuav) ) ) );

== matlab function sim_pos_dist_obs_tcyb/cal abs 44 ==
  data: x input; y output
function y = fcn(x)
y = abs(x(:));

== matlab function sim_pos_dist_obs_tcyb/cal abs 45 ==
  data: x input; y output
function y = fcn(x)
y = abs(x(:));

== matlab function sim_pos_dist_obs_tcyb/cal abs 46 ==
  data: x input; y output
function y = fcn(x)
y = abs(x(:));

== matlab function sim_pos_dist_obs_tcyb/cal abs 47 ==
  data: x input; y output
function y = fcn(x)
y = abs(x(:));

== matlab function sim_pos_dist_obs_tcyb/cal abs 48 ==
  data: x input; y output
function y = fcn(x)
y = abs(x(:));

== matlab function sim_pos_dist_obs_tcyb/cal abs 49 ==
  data: x input; y output
function y = fcn(x)
y = abs(x(:));

== matlab function sim_pos_dist_obs_tcyb/cal abs 50 ==
  data: x input; y output
function y = fcn(x)
y = abs(x(:));

== matlab function sim_pos_dist_obs_tcyb/cal abs 51 ==
  data: x input; y output
function y = fcn(x)
y = abs(x(:));

== matlab function sim_pos_dist_obs_tcyb/cal abs 52 ==
  data: x input; y output
function y = fcn(x)
y = abs(x(:));

== matlab function sim_pos_dist_obs_tcyb/cal abs 53 ==
  data: x input; y output
function y = fcn(x)
y = abs(x(:));

== matlab function sim_pos_dist_obs_tcyb/cal abs 54 ==
  data: x input; y output
function y = fcn(x)
y = abs(x(:));

== matlab function sim_pos_dist_obs_tcyb/cal abs 55 ==
  data: x input; y output
function y = fcn(x)
y = abs(x(:));

== matlab function sim_pos_dist_obs_tcyb/cal abs 56 ==
  data: x input; y output
function y = fcn(x)
y = abs(x(:));

== matlab function sim_pos_dist_obs_tcyb/cal abs 57 ==
  data: x input; y output
function y = fcn(x)
y = abs(x(:));

== matlab function sim_pos_dist_obs_tcyb/cal abs 58 ==
  data: x input; y output
function y = fcn(x)
y = abs(x(:));

== matlab function sim_pos_dist_obs_tcyb/cal abs 59 ==
  data: x input; y output
function y = fcn(x)
y = abs(x(:));

== matlab function sim_pos_dist_obs_tcyb/choose ksi_est_err 3 ==
  data: x input; y output
function y = fcn(x)
iiuav = 2;
y = x(:,iiuav);

== matlab function sim_pos_dist_obs_tcyb/cal abs 60 ==
  data: x input; y output
function y = fcn(x)
y = abs(x(:));

== matlab function sim_pos_dist_obs_tcyb/cal lumped observation error agent 1 ==
  data: wij input; w0 input; ksi_d_est_vec input; ksi0 input; delta_ksi_vec input; eta_d_est_vec input; ksi_est_err_tilt_1 output; eta0 input; delta_eta_vec input; eta_est_err_tilt_1 output
function [ksi_est_err_tilt_1, eta_est_err_tilt_1]  = fcn(wij, w0, ksi_d_est_vec, ksi0, delta_ksi_vec, eta_d_est_vec, eta0, delta_eta_vec)
%%%% 计算跟随者期望速度分布式观测器误差
iiuav = 1;
ksi_est_err_tilt_1 = w0(iiuav, iiuav) * (ksi_d_est_vec(:,iiuav) - ksi0(:) - delta_ksi_vec(:,iiuav));
eta_est_err_tilt_1 = w0(iiuav, iiuav) * (eta_d_est_vec(:,iiuav) - eta0(:) - delta_eta_vec(:,iiuav));
for jjuav = 1:5
    ksi_est_err_tilt_1 = ksi_est_err_tilt_1 + ...
                                        wij(iiuav, jjuav) * ((ksi_d_est_vec(:,iiuav) - delta_ksi_vec(:,iiuav)) - (ksi_d_est_vec(:,jjuav) - delta_ksi_vec(:,jjuav)));
    eta_est_err_tilt_1 = eta_est_err_tilt_1 + ...
                                        wij(iiuav, jjuav) * ((eta_d_est_vec(:,iiuav) - delta_eta_vec(:,iiuav)) - (eta_d_est_vec(:,jjuav) - delta_eta_vec(:,jjuav)));
end

== matlab function sim_pos_dist_obs_tcyb/cal lumped observation error agent 2 ==
  data: wij input; w0 input; ksi_d_est_vec input; ksi0 input; delta_ksi_vec input; eta_d_est_vec input; ksi_est_err_tilt_2 output; eta0 input; delta_eta_vec input; eta_est_err_tilt_2 output
function [ksi_est_err_tilt_2, eta_est_err_tilt_2]  = fcn(wij, w0, ksi_d_est_vec, ksi0, delta_ksi_vec, eta_d_est_vec, eta0, delta_eta_vec)
%%%% 计算跟随者期望速度分布式观测器误差
iiuav = 2;
ksi_est_err_tilt_2 = w0(iiuav, iiuav) * (ksi_d_est_vec(:,iiuav) - ksi0(:) - delta_ksi_vec(:,iiuav));
eta_est_err_tilt_2 = w0(iiuav, iiuav) * (eta_d_est_vec(:,iiuav) - eta0(:) - delta_eta_vec(:,iiuav));
for jjuav = 1:5
    ksi_est_err_tilt_2 = ksi_est_err_tilt_2 + ...
                                        wij(iiuav, jjuav) * ((ksi_d_est_vec(:,iiuav) - delta_ksi_vec(:,iiuav)) - (ksi_d_est_vec(:,jjuav) - delta_ksi_vec(:,jjuav)));
    eta_est_err_tilt_2 = eta_est_err_tilt_2 + ...
                                        wij(iiuav, jjuav) * ((eta_d_est_vec(:,iiuav) - delta_eta_vec(:,iiuav)) - (eta_d_est_vec(:,jjuav) - delta_eta_vec(:,jjuav)));
end

== matlab function sim_pos_dist_obs_tcyb/cal lumped observation error agent 3 ==
  data: wij input; w0 input; ksi_d_est_vec input; ksi0 input; delta_ksi_vec input; eta_d_est_vec input; ksi_est_err_tilt_3 output; eta0 input; delta_eta_vec input; eta_est_err_tilt_3 output
function [ksi_est_err_tilt_3, eta_est_err_tilt_3]  = fcn(wij, w0, ksi_d_est_vec, ksi0, delta_ksi_vec, eta_d_est_vec, eta0, delta_eta_vec)
%%%% 计算跟随者期望速度分布式观测器误差
iiuav = 3;
ksi_est_err_tilt_3 = w0(iiuav, iiuav) * (ksi_d_est_vec(:,iiuav) - ksi0(:) - delta_ksi_vec(:,iiuav));
eta_est_err_tilt_3 = w0(iiuav, iiuav) * (eta_d_est_vec(:,iiuav) - eta0(:) - delta_eta_vec(:,iiuav));
for jjuav = 1:5
    ksi_est_err_tilt_3 = ksi_est_err_tilt_3 + ...
                                        wij(iiuav, jjuav) * ((ksi_d_est_vec(:,iiuav) - delta_ksi_vec(:,iiuav)) - (ksi_d_est_vec(:,jjuav) - delta_ksi_vec(:,jjuav)));
    eta_est_err_tilt_3 = eta_est_err_tilt_3 + ...
                                        wij(iiuav, jjuav) * ((eta_d_est_vec(:,iiuav) - delta_eta_vec(:,iiuav)) - (eta_d_est_vec(:,jjuav) - delta_eta_vec(:,jjuav)));
end

== matlab function sim_pos_dist_obs_tcyb/cal lumped observation error agent 4 ==
  data: wij input; w0 input; ksi_d_est_vec input; ksi0 input; delta_ksi_vec input; eta_d_est_vec input; ksi_est_err_tilt_4 output; eta0 input; delta_eta_vec input; eta_est_err_tilt_4 output
function [ksi_est_err_tilt_4, eta_est_err_tilt_4]  = fcn(wij, w0, ksi_d_est_vec, ksi0, delta_ksi_vec, eta_d_est_vec, eta0, delta_eta_vec)
%%%% 计算跟随者期望速度分布式观测器误差
iiuav = 4;
ksi_est_err_tilt_4 = w0(iiuav, iiuav) * (ksi_d_est_vec(:,iiuav) - ksi0(:) - delta_ksi_vec(:,iiuav));
eta_est_err_tilt_4 = w0(iiuav, iiuav) * (eta_d_est_vec(:,iiuav) - eta0(:) - delta_eta_vec(:,iiuav));
for jjuav = 1:5
    ksi_est_err_tilt_4 = ksi_est_err_tilt_4 + ...
                                        wij(iiuav, jjuav) * ((ksi_d_est_vec(:,iiuav) - delta_ksi_vec(:,iiuav)) - (ksi_d_est_vec(:,jjuav) - delta_ksi_vec(:,jjuav)));
    eta_est_err_tilt_4 = eta_est_err_tilt_4 + ...
                                        wij(iiuav, jjuav) * ((eta_d_est_vec(:,iiuav) - delta_eta_vec(:,iiuav)) - (eta_d_est_vec(:,jjuav) - delta_eta_vec(:,jjuav)));
end

== matlab function sim_pos_dist_obs_tcyb/choose ksi_est_err 4 ==
  data: x input; y output
function y = fcn(x)
iiuav = 2;
y = x(:,iiuav);

== matlab function sim_pos_dist_obs_tcyb/cal lumped observation error agent 5 ==
  data: wij input; w0 input; ksi_d_est_vec input; ksi0 input; delta_ksi_vec input; eta_d_est_vec input; ksi_est_err_tilt_5 output; eta0 input; delta_eta_vec input; eta_est_err_tilt_5 output
function [ksi_est_err_tilt_5, eta_est_err_tilt_5]  = fcn(wij, w0, ksi_d_est_vec, ksi0, delta_ksi_vec, eta_d_est_vec, eta0, delta_eta_vec)
%%%% 计算跟随者期望速度分布式观测器误差
iiuav = 5;
ksi_est_err_tilt_5 = w0(iiuav, iiuav) * (ksi_d_est_vec(:,iiuav) - ksi0(:) - delta_ksi_vec(:,iiuav));
eta_est_err_tilt_5 = w0(iiuav, iiuav) * (eta_d_est_vec(:,iiuav) - eta0(:) - delta_eta_vec(:,iiuav));
for jjuav = 1:5
    ksi_est_err_tilt_5 = ksi_est_err_tilt_5 + ...
                                        wij(iiuav, jjuav) * ((ksi_d_est_vec(:,iiuav) - delta_ksi_vec(:,iiuav)) - (ksi_d_est_vec(:,jjuav) - delta_ksi_vec(:,jjuav)));
    eta_est_err_tilt_5 = eta_est_err_tilt_5 + ...
                                        wij(iiuav, jjuav) * ((eta_d_est_vec(:,iiuav) - delta_eta_vec(:,iiuav)) - (eta_d_est_vec(:,jjuav) - delta_eta_vec(:,jjuav)));
end

== matlab function sim_pos_dist_obs_tcyb/cal position estimate error ==
  data: ksi_d_est_vec input; ksi_est_err output; ksi0 input; delta_ksi_vec input
function ksi_est_err  = fcn(ksi_d_est_vec, ksi0, delta_ksi_vec)
%%%% 计算跟随者期望位置分布式观测器误差
ksi_est_err = ksi_d_est_vec - repmat(ksi0, 1, 5) - delta_ksi_vec;

== matlab function sim_pos_dist_obs_tcyb/cal theta_eta_est_err_tilt agent 1 ==
  data: alfa_theta input; eta_est_err_squ_1_node_1 input; theta_eta_est_err_tilt_1_1 output; eta_est_err_squ_2_node_1 input; eta_est_err_tilt_vec input; theta_eta_est_err_tilt_2_1 output
function [theta_eta_est_err_tilt_1_1, theta_eta_est_err_tilt_2_1] = fcn(alfa_theta, eta_est_err_squ_1_node_1, eta_est_err_squ_2_node_1, eta_est_err_tilt_vec)
%%%% 计算平滑递增函数
iiuav = 1;
theta_eta_est_err_tilt_1_1 = eta_est_err_squ_1_node_1(:) .* ( -1 + 2 ./ ( 1 + exp( -alfa_theta .* eta_est_err_tilt_vec(:,iiuav) ) ) );
theta_eta_est_err_tilt_2_1 = eta_est_err_squ_2_node_1(:) .* ( -1 + 2 ./ ( 1 + exp( -alfa_theta .* eta_est_err_tilt_vec(:,iiuav) ) ) );

== matlab function sim_pos_dist_obs_tcyb/cal theta_eta_est_err_tilt agent 2 ==
  data: alfa_theta input; eta_est_err_squ_1_node_2 input; theta_eta_est_err_tilt_1_2 output; eta_est_err_squ_2_node_2 input; eta_est_err_tilt_vec input; theta_eta_est_err_tilt_2_2 output
function [theta_eta_est_err_tilt_1_2, theta_eta_est_err_tilt_2_2] = fcn(alfa_theta, eta_est_err_squ_1_node_2, eta_est_err_squ_2_node_2, eta_est_err_tilt_vec)
%%%% 计算平滑递增函数
iiuav = 2;
theta_eta_est_err_tilt_1_2 = eta_est_err_squ_1_node_2(:) .* ( -1 + 2 ./ ( 1 + exp( -alfa_theta .* eta_est_err_tilt_vec(:,iiuav) ) ) );
theta_eta_est_err_tilt_2_2 = eta_est_err_squ_2_node_2(:) .* ( -1 + 2 ./ ( 1 + exp( -alfa_theta .* eta_est_err_tilt_vec(:,iiuav) ) ) );

== matlab function sim_pos_dist_obs_tcyb/cal theta_eta_est_err_tilt agent 3 ==
  data: alfa_theta input; eta_est_err_squ_1_node_3 input; theta_eta_est_err_tilt_1_3 output; eta_est_err_squ_2_node_3 input; eta_est_err_tilt_vec input; theta_eta_est_err_tilt_2_3 output
function [theta_eta_est_err_tilt_1_3, theta_eta_est_err_tilt_2_3] = fcn(alfa_theta, eta_est_err_squ_1_node_3, eta_est_err_squ_2_node_3, eta_est_err_tilt_vec)
%%%% 计算平滑递增函数
iiuav = 3;
theta_eta_est_err_tilt_1_3 = eta_est_err_squ_1_node_3(:) .* ( -1 + 2 ./ ( 1 + exp( -alfa_theta .* eta_est_err_tilt_vec(:,iiuav) ) ) );
theta_eta_est_err_tilt_2_3 = eta_est_err_squ_2_node_3(:) .* ( -1 + 2 ./ ( 1 + exp( -alfa_theta .* eta_est_err_tilt_vec(:,iiuav) ) ) );

== matlab function sim_pos_dist_obs_tcyb/cal theta_eta_est_err_tilt agent 4 ==
  data: alfa_theta input; eta_est_err_squ_1_node_4 input; theta_eta_est_err_tilt_1_4 output; eta_est_err_squ_2_node_4 input; eta_est_err_tilt_vec input; theta_eta_est_err_tilt_2_4 output
function [theta_eta_est_err_tilt_1_4, theta_eta_est_err_tilt_2_4] = fcn(alfa_theta, eta_est_err_squ_1_node_4, eta_est_err_squ_2_node_4, eta_est_err_tilt_vec)
%%%% 计算平滑递增函数
iiuav = 4;
theta_eta_est_err_tilt_1_4 = eta_est_err_squ_1_node_4(:) .* ( -1 + 2 ./ ( 1 + exp( -alfa_theta .* eta_est_err_tilt_vec(:,iiuav) ) ) );
theta_eta_est_err_tilt_2_4 = eta_est_err_squ_2_node_4(:) .* ( -1 + 2 ./ ( 1 + exp( -alfa_theta .* eta_est_err_tilt_vec(:,iiuav) ) ) );

== matlab function sim_pos_dist_obs_tcyb/cal theta_eta_est_err_tilt agent 5 ==
  data: alfa_theta input; eta_est_err_squ_1_node_5 input; theta_eta_est_err_tilt_1_5 output; eta_est_err_squ_2_node_5 input; eta_est_err_tilt_vec input; theta_eta_est_err_tilt_2_5 output
function [theta_eta_est_err_tilt_1_5, theta_eta_est_err_tilt_2_5] = fcn(alfa_theta, eta_est_err_squ_1_node_5, eta_est_err_squ_2_node_5, eta_est_err_tilt_vec)
%%%% 计算平滑递增函数
iiuav = 5;
theta_eta_est_err_tilt_1_5 = eta_est_err_squ_1_node_5(:) .* ( -1 + 2 ./ ( 1 + exp( -alfa_theta .* eta_est_err_tilt_vec(:,iiuav) ) ) );
theta_eta_est_err_tilt_2_5 = eta_est_err_squ_2_node_5(:) .* ( -1 + 2 ./ ( 1 + exp( -alfa_theta .* eta_est_err_tilt_vec(:,iiuav) ) ) );

== matlab function sim_pos_dist_obs_tcyb/trans to column2 ==
  data: x input; y output
function y = fcn(x)
y = x(:);

== matlab function sim_pos_dist_obs_tcyb/cal theta_ksi_est_err_tilt agent 1 ==
  data: alfa_theta input; ksi_est_err_squ_1_node_1 input; theta_ksi_est_err_tilt_1_1 output; ksi_est_err_squ_2_node_1 input; ksi_est_err_tilt_vec input; theta_ksi_est_err_tilt_2_1 output
function [theta_ksi_est_err_tilt_1_1, theta_ksi_est_err_tilt_2_1] = fcn(alfa_theta, ksi_est_err_squ_1_node_1, ksi_est_err_squ_2_node_1, ksi_est_err_tilt_vec)
%%%% 计算平滑递增函数
iiuav = 1;
theta_ksi_est_err_tilt_1_1 = ksi_est_err_squ_1_node_1(:) .* ( -1 + 2 ./ ( 1 + exp( -alfa_theta .* ksi_est_err_tilt_vec(:,iiuav) ) ) );
theta_ksi_est_err_tilt_2_1 = ksi_est_err_squ_2_node_1(:) .* ( -1 + 2 ./ ( 1 + exp( -alfa_theta .* ksi_est_err_tilt_vec(:,iiuav) ) ) );

== matlab function sim_pos_dist_obs_tcyb/cal theta_ksi_est_err_tilt agent 2 ==
  data: alfa_theta input; ksi_est_err_squ_1_node_2 input; theta_ksi_est_err_tilt_1_2 output; ksi_est_err_squ_2_node_2 input; ksi_est_err_tilt_vec input; theta_ksi_est_err_tilt_2_2 output
function [theta_ksi_est_err_tilt_1_2, theta_ksi_est_err_tilt_2_2] = fcn(alfa_theta, ksi_est_err_squ_1_node_2, ksi_est_err_squ_2_node_2, ksi_est_err_tilt_vec)
%%%% 计算平滑递增函数
iiuav = 2;
theta_ksi_est_err_tilt_1_2 = ksi_est_err_squ_1_node_2(:) .* ( -1 + 2 ./ ( 1 + exp( -alfa_theta .* ksi_est_err_tilt_vec(:,iiuav) ) ) );
theta_ksi_est_err_tilt_2_2 = ksi_est_err_squ_2_node_2(:) .* ( -1 + 2 ./ ( 1 + exp( -alfa_theta .* ksi_est_err_tilt_vec(:,iiuav) ) ) );

== matlab function sim_pos_dist_obs_tcyb/cal theta_ksi_est_err_tilt agent 3 ==
  data: alfa_theta input; ksi_est_err_squ_1_node_3 input; theta_ksi_est_err_tilt_1_3 output; ksi_est_err_squ_2_node_3 input; ksi_est_err_tilt_vec input; theta_ksi_est_err_tilt_2_3 output
function [theta_ksi_est_err_tilt_1_3, theta_ksi_est_err_tilt_2_3] = fcn(alfa_theta, ksi_est_err_squ_1_node_3, ksi_est_err_squ_2_node_3, ksi_est_err_tilt_vec)
%%%% 计算平滑递增函数
iiuav = 3;
theta_ksi_est_err_tilt_1_3 = ksi_est_err_squ_1_node_3(:) .* ( -1 + 2 ./ ( 1 + exp( -alfa_theta .* ksi_est_err_tilt_vec(:,iiuav) ) ) );
theta_ksi_est_err_tilt_2_3 = ksi_est_err_squ_2_node_3(:) .* ( -1 + 2 ./ ( 1 + exp( -alfa_theta .* ksi_est_err_tilt_vec(:,iiuav) ) ) );

== matlab function sim_pos_dist_obs_tcyb/cal theta_ksi_est_err_tilt agent 4 ==
  data: alfa_theta input; ksi_est_err_squ_1_node_4 input; theta_ksi_est_err_tilt_1_4 output; ksi_est_err_squ_2_node_4 input; ksi_est_err_tilt_vec input; theta_ksi_est_err_tilt_2_4 output
function [theta_ksi_est_err_tilt_1_4, theta_ksi_est_err_tilt_2_4] = fcn(alfa_theta, ksi_est_err_squ_1_node_4, ksi_est_err_squ_2_node_4, ksi_est_err_tilt_vec)
%%%% 计算平滑递增函数
iiuav = 4;
theta_ksi_est_err_tilt_1_4 = ksi_est_err_squ_1_node_4(:) .* ( -1 + 2 ./ ( 1 + exp( -alfa_theta .* ksi_est_err_tilt_vec(:,iiuav) ) ) );
theta_ksi_est_err_tilt_2_4 = ksi_est_err_squ_2_node_4(:) .* ( -1 + 2 ./ ( 1 + exp( -alfa_theta .* ksi_est_err_tilt_vec(:,iiuav) ) ) );

== matlab function sim_pos_dist_obs_tcyb/cal theta_ksi_est_err_tilt agent 5 ==
  data: alfa_theta input; ksi_est_err_squ_1_node_5 input; theta_ksi_est_err_tilt_1_5 output; ksi_est_err_squ_2_node_5 input; ksi_est_err_tilt_vec input; theta_ksi_est_err_tilt_2_5 output
function [theta_ksi_est_err_tilt_1_5, theta_ksi_est_err_tilt_2_5] = fcn(alfa_theta, ksi_est_err_squ_1_node_5, ksi_est_err_squ_2_node_5, ksi_est_err_tilt_vec)
%%%% 计算平滑递增函数
iiuav = 5;
theta_ksi_est_err_tilt_1_5 = ksi_est_err_squ_1_node_5(:) .* ( -1 + 2 ./ ( 1 + exp( -alfa_theta .* ksi_est_err_tilt_vec(:,iiuav) ) ) );
theta_ksi_est_err_tilt_2_5 = ksi_est_err_squ_2_node_5(:) .* ( -1 + 2 ./ ( 1 + exp( -alfa_theta .* ksi_est_err_tilt_vec(:,iiuav) ) ) );

== matlab function sim_pos_dist_obs_tcyb/cal velocity estimate error ==
  data: eta_d_est_vec input; eta_est_err output; eta0 input; delta_eta_vec input
function eta_est_err  = fcn(eta_d_est_vec, eta0, delta_eta_vec)
%%%% 计算跟随者期望速度分布式观测器误差
eta_est_err = eta_d_est_vec - repmat(eta0, 1, 5) - delta_eta_vec;

== matlab function sim_pos_dist_obs_tcyb/trans to column3 ==
  data: x input; y output
function y = fcn(x)
y = x(:);

== matlab function sim_pos_dist_obs_tcyb/choose eta_est_err_tilt 1 ==
  data: x input; y output
function y = fcn(x)
iiuav = 1;
y = x(:,iiuav);

== matlab function sim_pos_dist_obs_tcyb/choose eta_est_err_tilt 10 ==
  data: x input; y output
function y = fcn(x)
iiuav = 5;
y = x(:,iiuav);

== matlab function sim_pos_dist_obs_tcyb/choose eta_est_err_tilt 11 ==
  data: x input; y output
function y = fcn(x)
iiuav = 1;
y = x(:,iiuav);

== matlab function sim_pos_dist_obs_tcyb/choose eta_est_err_tilt 12 ==
  data: x input; y output
function y = fcn(x)
iiuav = 5;
y = x(:,iiuav);

== matlab function sim_pos_dist_obs_tcyb/choose eta_est_err_tilt 13 ==
  data: x input; y output
function y = fcn(x)
iiuav = 1;
y = x(:,iiuav);

== matlab function sim_pos_dist_obs_tcyb/choose eta_est_err_tilt 14 ==
  data: x input; y output
function y = fcn(x)
iiuav = 2;
y = x(:,iiuav);

== matlab function sim_pos_dist_obs_tcyb/choose eta_est_err_tilt 15 ==
  data: x input; y output
function y = fcn(x)
iiuav = 2;
y = x(:,iiuav);

== matlab function sim_pos_dist_obs_tcyb/choose eta_est_err_tilt 16 ==
  data: x input; y output
function y = fcn(x)
iiuav = 3;
y = x(:,iiuav);

== matlab function sim_pos_dist_obs_tcyb/choose eta_est_err_tilt 17 ==
  data: x input; y output
function y = fcn(x)
iiuav = 3;
y = x(:,iiuav);

== matlab function sim_pos_dist_obs_tcyb/choose eta_est_err_tilt 18 ==
  data: x input; y output
function y = fcn(x)
iiuav = 4;
y = x(:,iiuav);

== matlab function sim_pos_dist_obs_tcyb/cal abs 5 ==
  data: x input; y output
function y = fcn(x)
y = abs(x(:));

== matlab function sim_pos_dist_obs_tcyb/choose eta_est_err_tilt 19 ==
  data: x input; y output
function y = fcn(x)
iiuav = 4;
y = x(:,iiuav);

== matlab function sim_pos_dist_obs_tcyb/choose eta_est_err_tilt 2 ==
  data: x input; y output
function y = fcn(x)
iiuav = 1;
y = x(:,iiuav);

== matlab function sim_pos_dist_obs_tcyb/choose eta_est_err_tilt 20 ==
  data: x input; y output
function y = fcn(x)
iiuav = 5;
y = x(:,iiuav);

== matlab function sim_pos_dist_obs_tcyb/choose eta_est_err_tilt 3 ==
  data: x input; y output
function y = fcn(x)
iiuav = 2;
y = x(:,iiuav);

== matlab function sim_pos_dist_obs_tcyb/choose eta_est_err_tilt 4 ==
  data: x input; y output
function y = fcn(x)
iiuav = 2;
y = x(:,iiuav);

== matlab function sim_pos_dist_obs_tcyb/choose eta_est_err_tilt 5 ==
  data: x input; y output
function y = fcn(x)
iiuav = 3;
y = x(:,iiuav);

== matlab function sim_pos_dist_obs_tcyb/choose eta_est_err_tilt 6 ==
  data: x input; y output
function y = fcn(x)
iiuav = 3;
y = x(:,iiuav);
